simulink model "testsystem2"  (Simulink 8.5)
settings: Solver=ode23tb  SolverMode=SingleTasking  StartTime=0.0  StopTime=0.1  RelTol=1e-3  AbsTol=1e-6
libraries: powerlib x43, powerlib_extras x1
settings Model: Creator=PC  LastModifiedBy=PC  ExtModeTrigMode=oneshot  ExtModeArmWhenConnect=off
settings DataIOCC: LimitDataPoints=off
settings OptimizationCC: BlockReduction=off  BooleanDataType=off  ExpressionDepthLimit=128
settings DebuggingCC: SaveWithParameterizedLinksMsg=none  SignalResolutionControl=TryResolveAllWithWarning  MultiTaskDSMMsg=warning  MultiTaskCondExecSysMsg=none  FcnCallInpInsideContextMsg=EnableAllAsError  StateNameClashWarn=none  StrictBusMsg=None
settings HardwareCC: TargetUnknown=on

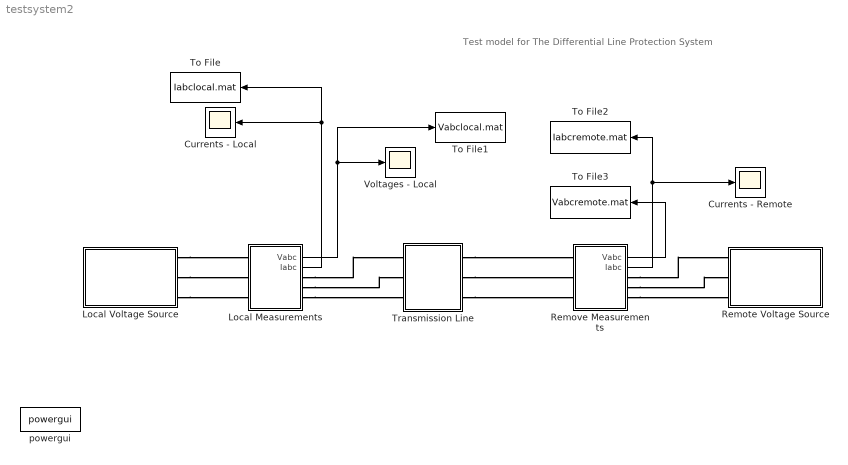
== system testsystem2 ==
  note: Test model for The Differential Line Protection System
  Currents - Local : Scope
      settings: TickLabels=on  YMin=-0.3  YMax=0.2
  Currents - Remote : Scope
      settings: TickLabels=on  YMin=-0.3  YMax=0.3
  Local Measurements : Subsystem  mask{VT=2000, CT=100}
      mask prompts: VT "VT ratio"; CT "CT ratio"
  Local Voltage Source : Subsystem  mask(3-phase inductive source - Ungrounded neutral){V=194367, Phi=10, F=60, R=3.4878, L=0.1323}
      mask prompts: V "Voltage magnitude (V) :"; Phi "Phase angle of phase A (Degrees) :"; F "Frequency (Hz) :"; R "Source resistance (Ohms):"; L "Source inductance (H) :"
      mask init:
      | a=R;b=L;c=inf;
      | short_x =[0,150];
      | short_y =[0,0];
      | 
      | resistor_x = [0 30,30,38,53,68,83,98,113,120,120,150];
      | resistor_y = [0,0,0,25,-25,25,-25,25,-25,0,0,0];
      | 
      | inductor_x = [150,173,173,174,178,184,190,197,202,205,206,204,201,201,197,196,198,201,207,214,220,225,229,229,227,224,224,220,219,221,225,230,237,243,249,252,253,251,247,247,244,243,244,248,254,260,267,272,275,276,276,300];
      | 
      | inductor_y = [0,0,1,11,19,24,25,23,17,8,-2,-12,-18,-18,-9,1,11,19,24,25,23,17,8,-2,-12,-18,-18,-9,1,11,19,24,25,23,17,8,-2,-12,-18,-18,-9,1, 11,19,24,25,23,17,8,0,0,0];
      | 
      | capacitor_x1 = [300 360 360 360];
      | capacitor_y1 = [0 0 25 -25];
      | capacitor_x2 = [390 390 390 450];
      | capacitor_y2 = [25,-25,0,0];
      | if a~=0
      | 	s1=resistor_x;
      | 	s2=resistor_y;
      | else
      | 	s1=short_x;
      | 	s2=short_y;
      | end
      | 
      | if b~=0
      | 	s3=inductor_x;
      | 	s4=inductor_y;
      | else
      | 	s3=short_x+150;
      | 	s4=short_y;
      | end
      | 
      | s5=[];
      | s6=[];
      | s7=[];
      | s8=[];
      mask Display: plot(-170,-60,360,60,s1,s2,s3,s4,s5,s6,s7,s8, [0,9,18,24,29,30,29,24,18,9,0,-9,-18,-24,-29,-30,-29,-24,-18,-9,0]*1.5-45,  [30,29,24,18,9,0,-9,-18,-24,-29,-30,-29,-24,-18,-9,0,9,18,24,29,30]*0.8,[-150,-90],[0,0],[-150,-150],[-20,20],[-165,-165],[-15,15],[-180,-180],[-10,10])
  "Remote Voltage Source " : Subsystem  mask(3-phase inductive source - Ungrounded neutral){V=194367, Phi=0, F=60, R=3.4878, L=0.1323}
      mask prompts: V "Voltage magnitude (V) :"; Phi "Phase angle of phase A (Degrees) :"; F "Frequency (Hz) :"; R "Source resistance (Ohms):"; L "Source inductance (H) :"
      mask init: same as testsystem2/Local Voltage Source
      mask Display: plot(-170,-60,360,60,s1,s2,s3,s4,s5,s6,s7,s8, [0,9,18,24,29,30,29,24,18,9,0,-9,-18,-24,-29,-30,-29,-24,-18,-9,0]*1.5-45,  [30,29,24,18,9,0,-9,-18,-24,-29,-30,-29,-24,-18,-9,0,9,18,24,29,30]*0.8,[-150,-90],[0,0],[-150,-150],[-20,20],[-165,-165],[-15,15],[-180,-180],[-10,10])
  Remove Measurements : Subsystem  mask{VT=2000, CT=100}
      mask prompts: VT "VT ratio"; CT "CT ratio"
  To File : ToFile  Filename=Iabclocal.mat  MatrixName=Iabcl
  To File1 : ToFile  Filename=Vabclocal.mat  MatrixName=Vabc
  To File2 : ToFile  Filename=Iabcremote.mat  MatrixName=Iabcr
  To File3 : ToFile  Filename=Vabcremote.mat  MatrixName=Vabcr
  Transmission Line : Subsystem  mask(Teansmission line with fault){ff=60, rr=[0.0815 0.3666], ll=[2.1e-3 6.5e-3], cc=[31.6e-9 12.7e-9], length=40, faultLocation=0.5, faultType='C-A-G', faultR=0.01, faultTime=[9 10 11 12 13]}
      mask prompts: ff "Frequency used for R L C specification (Hz)"; rr "Resistance per unit length (Ohm/mile) [R1 R0]"; ll "Inductance per unit length (H/mile) [L1 L0]"; cc "Capacitance per unit length (F/mile) [C1 C0]"; length "Line length (mile)"; faultLocation "Fault location (p.u.) <0,1>"; faultType "Fault Type"; faultR "Fault Resistance per Phase (Ohm)"; faultTime "Fault time sequence (s) [C O C O C]"
      mask TypeOptions faultType: 'A-G' | 'B-G' | 'C-G' | 'B-C' | 'B-C-G' | 'C-A' | 'C-A-G' | 'A-B-C' | 'A-B-C-G'
  Voltages - Local : Scope
      settings: TickLabels=on  YMin=-450000  YMax=450000
  powergui : powerlib/powergui  SimulationMode=Continuous  SolverType=Tustin/Backward Euler (TBE)  SampleTime=0  frequency=60  SPID=off  DisableSnubberDevices=off  DisableRonSwitches=off  DisableVfSwitches=off  SwTol=0  DisplayEquations=off  Interpol=off  methode=off  Ts=0  FunctionMessages=off  echomessages=off  HookPort=off  EnableUseOfTLC=off  x0status=blocks  frequencyindice=60  Pbase=100e6  ErrMax=1e-4  Iterations=50  UnitsV=kV  UnitsW=MW  buscounter=0  RestoreLinks=warning  ResistiveCurrentMeasurement=off  Frange=[0:2:500]  Ylog=off  Xlog=on  ShowGrid=off  save=off  variable=ZData  structure=0  ZoomFFT=on  StartTime=0.0  cycles=1  DisplayStyle=1  fundamental=60  FreqAxis=off  MaxFrequency=1000  frequencyindicesteady=1  RmsSteady=1  display=off
  wires:
  Local Measurements/2(Iabc) -> Currents - Local/1, To File/1
  Local Measurements/1(Vabc) -> To File1/1, Voltages - Local/1
  Remove Measurements/2(Iabc) -> To File2/1, Currents - Remote/1
  Remove Measurements/1(Vabc) -> To File3/1
  connections:
  Local Voltage Source/RConn1 -- Local Measurements/LConn1
  Local Voltage Source/RConn2 -- Local Measurements/LConn2
  Local Voltage Source/RConn3 -- Local Measurements/LConn3
  Local Measurements/RConn1 -- Transmission Line/LConn1
  Local Measurements/RConn2 -- Transmission Line/LConn2
  Local Measurements/RConn3 -- Transmission Line/LConn3
  Transmission Line/RConn1 -- Remove Measurements/LConn1
  Transmission Line/RConn2 -- Remove Measurements/LConn2
  Transmission Line/RConn3 -- Remove Measurements/LConn3
  Remove Measurements/RConn1 -- "Remote Voltage Source "/RConn1
  Remove Measurements/RConn2 -- "Remote Voltage Source "/RConn2
  Remove Measurements/RConn3 -- "Remote Voltage Source "/RConn3

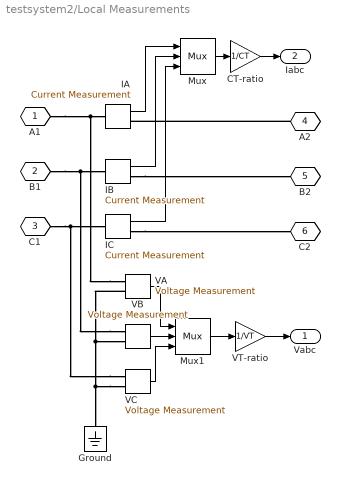
== system testsystem2/Local Measurements ==
  CT-ratio : Gain  Gain=1/CT  SaturateOnIntegerOverflow=on  OutDataTypeStr=Inherit: Same as input  ParamDataTypeStr=Inherit: Same as input
  Ground : powerlib/Elements/Ground  LConnTagsString=a
  IA : powerlib/Measurements/Current Measurement  PhasorSimulation=off  OutputType=Complex  PSBequivalent=0
  IB : powerlib/Measurements/Current Measurement  PhasorSimulation=off  OutputType=Complex  PSBequivalent=0
  IC : powerlib/Measurements/Current Measurement  PhasorSimulation=off  OutputType=Complex  PSBequivalent=0
  Mux : Mux  Inputs=3
  Mux1 : Mux  Inputs=3
  VA : powerlib/Measurements/Voltage Measurement  PhasorSimulation=off  OutputType=Complex  PSBequivalent=0
  VB : powerlib/Measurements/Voltage Measurement  PhasorSimulation=off  OutputType=Complex  PSBequivalent=0
  VC : powerlib/Measurements/Voltage Measurement  PhasorSimulation=off  OutputType=Complex  PSBequivalent=0
  VT-ratio : Gain  Gain=1/VT  SaturateOnIntegerOverflow=on  OutDataTypeStr=Inherit: Same as input  ParamDataTypeStr=Inherit: Same as input
  A1 : PMIOPort  Tag=PMCPort  Port=1  Side=Left
  B1 : PMIOPort  Tag=PMCPort  Port=2  Side=Left
  C1 : PMIOPort  Tag=PMCPort  Port=3  Side=Left
  A2 : PMIOPort  Tag=PMCPort  Port=4  Side=Right
  B2 : PMIOPort  Tag=PMCPort  Port=5  Side=Right
  C2 : PMIOPort  Tag=PMCPort  Port=6  Side=Right
  Vabc : Outport  InitialOutput=0
  Iabc : Outport  Port=2  InitialOutput=0
  wires:
  VC/1 -> Mux1/3
  VB/1 -> Mux1/2
  VA/1 -> Mux1/1
  CT-ratio/1 -> Iabc/1
  Mux/1 -> CT-ratio/1
  VT-ratio/1 -> Vabc/1
  Mux1/1 -> VT-ratio/1
  IA/1 -> Mux/1
  IB/1 -> Mux/2
  IC/1 -> Mux/3
  connections:
  IC/RConn1 -- C2/RConn1
  IB/RConn1 -- B2/RConn1
  A2/RConn1 -- IA/RConn1
  VC/LConn1 -- IC/LConn1 -- C1/RConn1
  VB/LConn1 -- IB/LConn1 -- B1/RConn1
  VA/LConn1 -- IA/LConn1 -- A1/RConn1
  VC/LConn2 -- Ground/LConn1 -- VB/LConn2 -- VA/LConn2

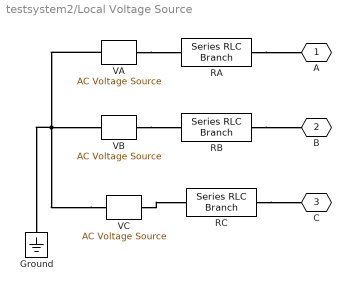
== system testsystem2/Local Voltage Source ==
  Ground : powerlib/Elements/Ground  LConnTagsString=a
  RA : powerlib/Elements/Series RLC Branch  LConnTagsString=__new0  RConnTagsString=__new0  BranchType=RL  Resistance=R  Inductance=L  SetiL0=off  InitialCurrent=0  Capacitance=1.0  Setx0=off  InitialVoltage=0  Measurements=None
  RB : powerlib/Elements/Series RLC Branch  LConnTagsString=__new0  RConnTagsString=__new0  BranchType=RL  Resistance=R  Inductance=L  SetiL0=off  InitialCurrent=0  Capacitance=1.0  Setx0=off  InitialVoltage=0  Measurements=None
  RC : powerlib/Elements/Series RLC Branch  LConnTagsString=__new0  RConnTagsString=__new0  BranchType=RL  Resistance=R  Inductance=L  SetiL0=off  InitialCurrent=0  Capacitance=1.0  Setx0=off  InitialVoltage=0  Measurements=None
  VA : powerlib/Electrical Sources/AC Voltage Source  Amplitude=V  Phase=Phi  Frequency=F  SampleTime=0  Measurements=None
  VB : powerlib/Electrical Sources/AC Voltage Source  Amplitude=V  Phase=Phi-120  Frequency=F  SampleTime=0  Measurements=None
  VC : powerlib/Electrical Sources/AC Voltage Source  Amplitude=V  Phase=Phi+120  Frequency=F  SampleTime=0  Measurements=None
  A : PMIOPort  Tag=PMCPort  Port=1  Side=Right
  B : PMIOPort  Tag=PMCPort  Port=2  Side=Right
  C : PMIOPort  Tag=PMCPort  Port=3  Side=Right
  connections:
  VC/LConn1 -- VA/LConn1 -- Ground/LConn1 -- VB/LConn1
  VA/RConn1 -- RA/LConn1
  VB/RConn1 -- RB/LConn1
  VC/RConn1 -- RC/LConn1
  RA/RConn1 -- A/RConn1
  RB/RConn1 -- B/RConn1
  RC/RConn1 -- C/RConn1

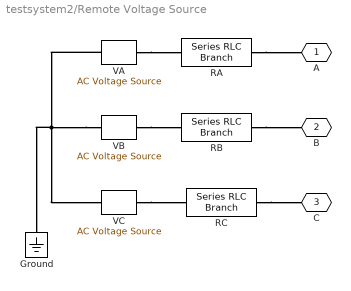
== system testsystem2/Remote Voltage Source  ==
  Ground : powerlib/Elements/Ground  LConnTagsString=a
  RA : powerlib/Elements/Series RLC Branch  LConnTagsString=__new0  RConnTagsString=__new0  BranchType=RL  Resistance=R  Inductance=L  SetiL0=off  InitialCurrent=0  Capacitance=1.0  Setx0=off  InitialVoltage=0  Measurements=None
  RB : powerlib/Elements/Series RLC Branch  LConnTagsString=__new0  RConnTagsString=__new0  BranchType=RL  Resistance=R  Inductance=L  SetiL0=off  InitialCurrent=0  Capacitance=1.0  Setx0=off  InitialVoltage=0  Measurements=None
  RC : powerlib/Elements/Series RLC Branch  LConnTagsString=__new0  RConnTagsString=__new0  BranchType=RL  Resistance=R  Inductance=L  SetiL0=off  InitialCurrent=0  Capacitance=1.0  Setx0=off  InitialVoltage=0  Measurements=None
  VA : powerlib/Electrical Sources/AC Voltage Source  Amplitude=V  Phase=Phi  Frequency=F  SampleTime=0  Measurements=Voltage
  VB : powerlib/Electrical Sources/AC Voltage Source  Amplitude=V  Phase=Phi-120  Frequency=F  SampleTime=0  Measurements=Voltage
  VC : powerlib/Electrical Sources/AC Voltage Source  Amplitude=V  Phase=Phi+120  Frequency=F  SampleTime=0  Measurements=None
  A : PMIOPort  Tag=PMCPort  Port=1  Side=Right
  B : PMIOPort  Tag=PMCPort  Port=2  Side=Right
  C : PMIOPort  Tag=PMCPort  Port=3  Side=Right
  connections:
  RC/RConn1 -- C/RConn1
  RB/RConn1 -- B/RConn1
  RA/RConn1 -- A/RConn1
  VC/RConn1 -- RC/LConn1
  VB/RConn1 -- RB/LConn1
  VA/RConn1 -- RA/LConn1
  VB/LConn1 -- Ground/LConn1 -- VA/LConn1 -- VC/LConn1

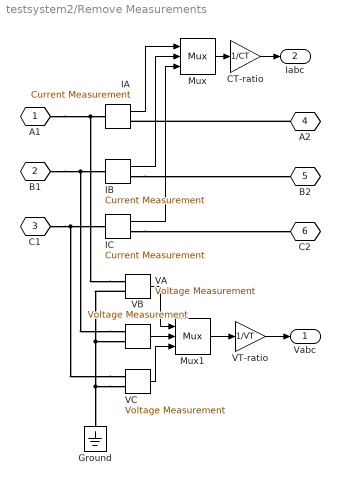
== system testsystem2/Remove Measurements ==
  CT-ratio : Gain  Gain=1/CT  SaturateOnIntegerOverflow=on  OutDataTypeStr=Inherit: Same as input  ParamDataTypeStr=Inherit: Same as input
  Ground : powerlib/Elements/Ground  LConnTagsString=a
  IA : powerlib/Measurements/Current Measurement  PhasorSimulation=off  OutputType=Complex  PSBequivalent=0
  IB : powerlib/Measurements/Current Measurement  PhasorSimulation=off  OutputType=Complex  PSBequivalent=0
  IC : powerlib/Measurements/Current Measurement  PhasorSimulation=off  OutputType=Complex  PSBequivalent=0
  Mux : Mux  Inputs=3
  Mux1 : Mux  Inputs=3
  VA : powerlib/Measurements/Voltage Measurement  PhasorSimulation=off  OutputType=Complex  PSBequivalent=0
  VB : powerlib/Measurements/Voltage Measurement  PhasorSimulation=off  OutputType=Complex  PSBequivalent=0
  VC : powerlib/Measurements/Voltage Measurement  PhasorSimulation=off  OutputType=Complex  PSBequivalent=0
  VT-ratio : Gain  Gain=1/VT  SaturateOnIntegerOverflow=on  OutDataTypeStr=Inherit: Same as input  ParamDataTypeStr=Inherit: Same as input
  A1 : PMIOPort  Tag=PMCPort  Port=1  Side=Left
  B1 : PMIOPort  Tag=PMCPort  Port=2  Side=Left
  C1 : PMIOPort  Tag=PMCPort  Port=3  Side=Left
  A2 : PMIOPort  Tag=PMCPort  Port=4  Side=Right
  B2 : PMIOPort  Tag=PMCPort  Port=5  Side=Right
  C2 : PMIOPort  Tag=PMCPort  Port=6  Side=Right
  Vabc : Outport  InitialOutput=0
  Iabc : Outport  Port=2  InitialOutput=0
  wires:
  VC/1 -> Mux1/3
  VB/1 -> Mux1/2
  VA/1 -> Mux1/1
  CT-ratio/1 -> Iabc/1
  Mux/1 -> CT-ratio/1
  VT-ratio/1 -> Vabc/1
  Mux1/1 -> VT-ratio/1
  IA/1 -> Mux/1
  IB/1 -> Mux/2
  IC/1 -> Mux/3
  connections:
  IC/RConn1 -- C2/RConn1
  IB/RConn1 -- B2/RConn1
  A2/RConn1 -- IA/RConn1
  VC/LConn1 -- IC/LConn1 -- C1/RConn1
  VB/LConn1 -- IB/LConn1 -- B1/RConn1
  VA/LConn1 -- IA/LConn1 -- A1/RConn1
  VC/LConn2 -- Ground/LConn1 -- VB/LConn2 -- VA/LConn2

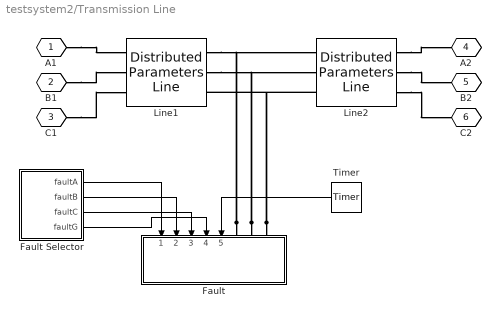
== system testsystem2/Transmission Line ==
  Fault : Subsystem
  Fault Selector : Subsystem
  Line1 : powerlib/Elements/Distributed Parameters Line  Phases=3  Frequency=ff  Resistance=rr  Inductance=ll  Capacitance=cc  Length=length*faultLocation  x1=[0 4.11902020198921e-010 134948.186782494 -205850.900154444;3.63428122191995e-005 4.0825381421406e-010 137755.779020702 -203982.723672073;7.26856244383991e-005 4.04528974006798e-010 140537.512818306 -202076.257143491;0.000109028436657599 4.00728198775092e-010 143292.866009928 -200131.858435729;0.000145371248876798 3.96852201970829e-010 146021.321382155 -198149.892536149;0.000181714061095998 3.92901711165905e-010 148722.36677062 -196130.731483934]  x2=[0 7.13787191208823e-010 132490.296601132 -209961.981117024;3.63428122191995e-005 7.1099393994792e-010 135354.443345949 -208127.093081486;7.26856244383991e-005 7.0806722644901e-010 138193.182410169 -206253.13705103;0.000109028436657599 7.05007600091929e-010 141005.98092783 -204340.46479007;0.000145371248876798 7.01815635205876e-010 143792.31090233 -202389.435330525;0.000181714061095998 6.98491930961609e-010 146551.649305534 -200400.414904433]  x3=[0 -6.76275058489345e-013 224.518563642735 -683.917970918056;3.63428122191995e-005 -6.09086881411019e-013 233.867501695858 -680.77776698083;7.26856244383991e-005 -5.41784371293034e-013 243.172539965284 -677.509772749958;0.000109028436657599 -4.74380161637757e-013 252.431931781791 -674.114601667833;0.000145371248876798 -4.068869050378e-013 261.643939044552 -670.592891049494;0.000181714061095998 -3.39317270800973e-013 270.806832547401 -666.945301962996]  x4=[0 3.07147625924859e-012 758.606072926325 -953.210303848756;3.63428122191995e-005 2.97855051235205e-012 771.594320195334 -942.727565252251;7.26856244383991e-005 2.88506565518036e-012 784.437729795524 -932.067865188679;0.000109028436657599 2.7910392359819e-012 797.133890862199 -921.233204613809;0.000145371248876798 2.69648890466286e-012 809.680420171009 -910.225617325636;0.000181714061095998 2.60143240947412e-012 822.074962585311 -899.047169582606]  x5=0.000181714061095998  V1=ones(3,3)  V2=ones(3,3)  I1=ones(3,3)  I2=ones(3,3)  nHarmo=1  Measurements=None
  Line2 : powerlib/Elements/Distributed Parameters Line  Phases=3  Frequency=ff  Resistance=rr  Inductance=ll  Capacitance=cc  Length=length*(1-faultLocation)  x1=[0 7.13787191208823e-010 132490.296601132 -209961.981117024;3.63428122191995e-005 7.1099393994792e-010 135354.443345949 -208127.093081486;7.26856244383991e-005 7.0806722644901e-010 138193.182410169 -206253.13705103;0.000109028436657599 7.05007600091929e-010 141005.98092783 -204340.46479007;0.000145371248876798 7.01815635205876e-010 143792.31090233 -202389.435330525;0.000181714061095998 6.98491930961609e-010 146551.649305534 -200400.414904433]  x2=[0 8.14266724137873e-010 129971.575736346 -213052.577881739;3.63428122191995e-005 8.05963056693762e-010 132878.301564795 -211251.907481799;7.26856244383991e-005 7.97508100149626e-010 135760.084514673 -209411.582521149;0.000109028436657599 7.88903441603976e-010 138616.383640156 -207531.94845124;0.000145371248876798 7.80150696256215e-010 141446.662779046 -205613.358102322;0.000181714061095998 7.71251507103443e-010 144250.390653414 -203656.171617215]  x3=[0 9.9534767771704e-012 277.764627888906 -689.162391337343;3.63428122191995e-005 9.96850032366961e-012 287.180419597183 -685.29219807324;7.26856244383991e-005 9.98165266102339e-012 296.542304036554 -681.293367101691;0.000109028436657599 9.99293132037755e-012 305.848523867077 -677.166649052061;0.000145371248876798 1.00023341845901e-011 315.097332197736 -672.912818559683;0.000181714061095998 1.00098594886287e-011 324.286992914355 -668.532674120445]  x4=[0 -7.55644004758007e-012 685.290952443927 -975.17875177988;3.63428122191995e-005 -7.56361063723915e-012 698.58705925878 -965.698404296413;7.26856244383991e-005 -7.56936144489117e-012 711.752032758518 -956.036783439102;0.000109028436657599 -7.57369139103938e-012 724.783401716979 -946.195702812072;0.000145371248876798 -7.57659966290005e-012 737.678719987202 -936.177009706237;0.000181714061095998 -7.57808571455506e-012 750.435566960599 -925.982584752539]  x5=0.000181714061095998  V1=ones(3,3)  V2=ones(3,3)  I1=ones(3,3)  I2=ones(3,3)  nHarmo=1  Measurements=None
  Timer : powerlib_extras/Control  Blocks/Timer  t=[0 faultTime]  e=[0 1 0 1 0 1]
  A1 : PMIOPort  Tag=PMCPort  Port=1  Side=Left
  B1 : PMIOPort  Tag=PMCPort  Port=2  Side=Left
  C1 : PMIOPort  Tag=PMCPort  Port=3  Side=Left
  A2 : PMIOPort  Tag=PMCPort  Port=4  Side=Right
  B2 : PMIOPort  Tag=PMCPort  Port=5  Side=Right
  C2 : PMIOPort  Tag=PMCPort  Port=6  Side=Right
  wires:
  Timer/1 -> Fault/5(Tfault)
  Fault Selector/4(faultG) -> Fault/4(faultG)
  Fault Selector/3(faultC) -> Fault/3(faultC)
  Fault Selector/2(faultB) -> Fault/2(faultB)
  Fault Selector/1(faultA) -> Fault/1(faultA)
  connections:
  Line2/RConn3 -- C2/RConn1
  Line2/RConn2 -- B2/RConn1
  Line2/RConn1 -- A2/RConn1
  C1/RConn1 -- Line1/LConn3
  B1/RConn1 -- Line1/LConn2
  A1/RConn1 -- Line1/LConn1
  Fault/LConn3 -- Line1/RConn3 -- Line2/LConn3
  Fault/LConn2 -- Line2/LConn2 -- Line1/RConn2
  Fault/LConn1 -- Line2/LConn1 -- Line1/RConn1

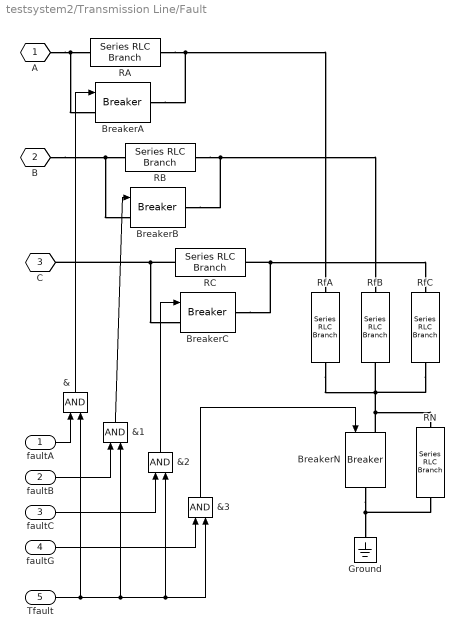
== system testsystem2/Transmission Line/Fault ==
  faultA : Inport
  faultB : Inport  Port=2
  faultC : Inport  Port=3
  faultG : Inport  Port=4
  Tfault : Inport  Port=5
  &{,1..3} (4 alike) : Logic
  BreakerA : powerlib/Elements/Breaker  InitialState=0  SwitchingTimes="[ 1/60  5/60 ]"  External=on  BreakerResistance=0.01  SnubberResistance=1e6  SnubberCapacitance=inf  Measurements=None  MoreParameters=off  NoBreakLoop=off
  BreakerB : powerlib/Elements/Breaker  InitialState=0  SwitchingTimes="[ 1/60  5/60 ]"  External=on  BreakerResistance=0.01  SnubberResistance=1e6  SnubberCapacitance=inf  Measurements=None  MoreParameters=off  NoBreakLoop=off
  BreakerC : powerlib/Elements/Breaker  InitialState=0  SwitchingTimes="[ 1/60  5/60 ]"  External=on  BreakerResistance=0.01  SnubberResistance=1e6  SnubberCapacitance=inf  Measurements=None  MoreParameters=off  NoBreakLoop=off
  BreakerN : powerlib/Elements/Breaker  InitialState=0  SwitchingTimes="[ 1/60  5/60 ]"  External=on  BreakerResistance=0.01  SnubberResistance=1e6  SnubberCapacitance=inf  Measurements=None  MoreParameters=off  NoBreakLoop=off
  Ground : powerlib/Elements/Ground  LConnTagsString=a
  RA : powerlib/Elements/Series RLC Branch  LConnTagsString=__new0  RConnTagsString=__new0  BranchType=R  Resistance=10000  Inductance=1e-3  SetiL0=off  InitialCurrent=0  Capacitance=1e-6  Setx0=off  InitialVoltage=0  Measurements=None
  RB : powerlib/Elements/Series RLC Branch  LConnTagsString=__new0  RConnTagsString=__new0  BranchType=R  Resistance=10000  Inductance=1e-3  SetiL0=off  InitialCurrent=0  Capacitance=1e-6  Setx0=off  InitialVoltage=0  Measurements=None
  RC : powerlib/Elements/Series RLC Branch  LConnTagsString=__new0  RConnTagsString=__new0  BranchType=R  Resistance=10000  Inductance=1e-3  SetiL0=off  InitialCurrent=0  Capacitance=1e-6  Setx0=off  InitialVoltage=0  Measurements=None
  RN : powerlib/Elements/Series RLC Branch  LConnTagsString=__new0  RConnTagsString=__new0  BranchType=R  Resistance=10000  Inductance=1e-3  SetiL0=off  InitialCurrent=0  Capacitance=1e-6  Setx0=off  InitialVoltage=0  Measurements=None
  RfA : powerlib/Elements/Series RLC Branch  LConnTagsString=__new0  RConnTagsString=__new0  BranchType=R  Resistance=faultR  Inductance=1e-3  SetiL0=off  InitialCurrent=0  Capacitance=1e-6  Setx0=off  InitialVoltage=0  Measurements=None
  RfB : powerlib/Elements/Series RLC Branch  LConnTagsString=__new0  RConnTagsString=__new0  BranchType=R  Resistance=faultR  Inductance=1e-3  SetiL0=off  InitialCurrent=0  Capacitance=1e-6  Setx0=off  InitialVoltage=0  Measurements=None
  RfC : powerlib/Elements/Series RLC Branch  LConnTagsString=__new0  RConnTagsString=__new0  BranchType=R  Resistance=faultR  Inductance=1e-3  SetiL0=off  InitialCurrent=0  Capacitance=1e-6  Setx0=off  InitialVoltage=0  Measurements=None
  A : PMIOPort  Tag=PMCPort  Port=1  Side=Left
  B : PMIOPort  Tag=PMCPort  Port=2  Side=Left
  C : PMIOPort  Tag=PMCPort  Port=3  Side=Left
  wires:
  faultA/1 -> &/1
  faultB/1 -> &1/1
  faultC/1 -> &2/1
  faultG/1 -> &3/1
  Tfault/1 -> &3/2, &2/2, &1/2, &/2
  &3/1 -> BreakerN/1
  &/1 -> BreakerA/1
  &1/1 -> BreakerB/1
  &2/1 -> BreakerC/1
  connections:
  B/RConn1 -- RB/LConn1 -- BreakerB/LConn1
  A/RConn1 -- BreakerA/LConn1 -- RA/LConn1
  RC/LConn1 -- C/RConn1 -- BreakerC/LConn1
  BreakerC/RConn1 -- RC/RConn1 -- RfC/LConn1
  RB/RConn1 -- RfB/LConn1 -- BreakerB/RConn1
  RA/RConn1 -- RfA/LConn1 -- BreakerA/RConn1
  BreakerN/LConn1 -- RN/LConn1 -- RfB/RConn1 -- RfA/RConn1 -- RfC/RConn1
  BreakerN/RConn1 -- Ground/LConn1 -- RN/RConn1

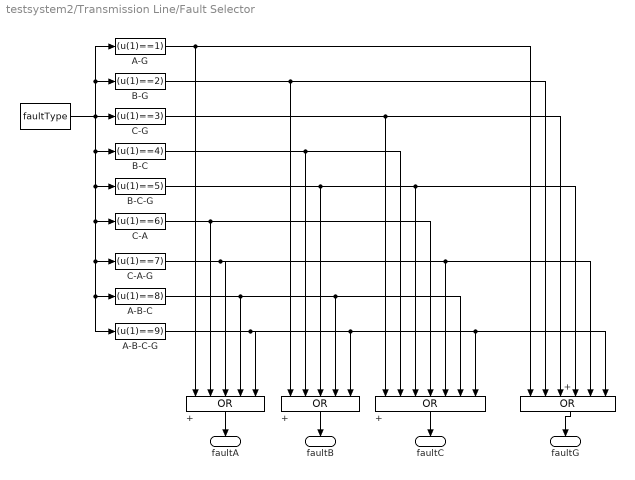
== system testsystem2/Transmission Line/Fault Selector ==
  "  " : Constant  Value=faultType
  "  +" : Logic  Operator=OR  Inputs=7
  " +" : Logic  Operator=OR  Inputs=5
  + : Logic  Operator=OR  Inputs=5
  "+ " : Logic  Operator=OR  Inputs=6
  A-B-C : Fcn  Expr=(u(1)==8)
  A-B-C-G : Fcn  Expr=(u(1)==9)
  A-G : Fcn  Expr=(u(1)==1)
  B-C : Fcn  Expr=(u(1)==4)
  B-C-G : Fcn  Expr=(u(1)==5)
  B-G : Fcn  Expr=(u(1)==2)
  C-A : Fcn  Expr=(u(1)==6)
  C-A-G : Fcn  Expr=(u(1)==7)
  C-G : Fcn  Expr=(u(1)==3)
  faultA : Outport  InitialOutput=0
  faultB : Outport  Port=2  InitialOutput=0
  faultC : Outport  Port=3  InitialOutput=0
  faultG : Outport  Port=4  InitialOutput=0
  wires:
  "  "/1 -> C-G/1, A-G/1, B-G/1, B-C/1, C-A/1, C-A-G/1, A-B-C/1, A-B-C-G/1, B-C-G/1
  +/1 -> faultA/1
  " +"/1 -> faultB/1
  "  +"/1 -> faultC/1
  "+ "/1 -> faultG/1
  A-G/1 -> "+ "/1, +/1
  C-A/1 -> "  +"/4, +/2
  B-G/1 -> " +"/1, "+ "/2
  B-C/1 -> "  +"/2, " +"/2
  B-C-G/1 -> "  +"/3, "+ "/4, " +"/3
  C-G/1 -> "  +"/1, "+ "/3
  C-A-G/1 -> "  +"/5, "+ "/5, +/3
  A-B-C-G/1 -> " +"/5, "  +"/7, "+ "/6, +/5
  A-B-C/1 -> " +"/4, "  +"/6, +/4
